simulink model "cont"  (R2017b)
settings: Solver=ode4  StartTime=0.0  StopTime=20  FixedStep=0.0001  RelTol=1e-3
settings Model: Creator=user  LastModifiedBy=user

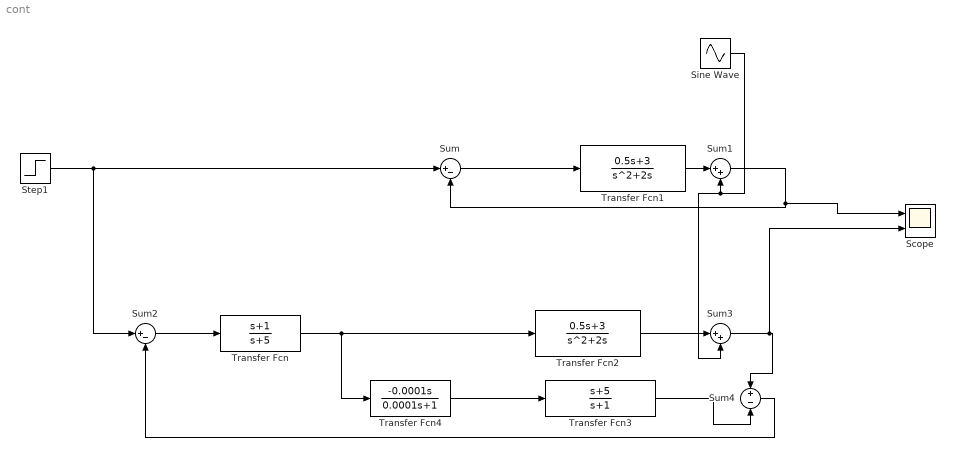
== system cont ==
  Scope : Scope  NumInputPorts=2
  Sine Wave : Sin  Amplitude=0.1  Frequency=10  Phase=2.7  SampleTime=0
  Step1 : Step  Time=0  SampleTime=0
  Sum : Sum  Inputs=|+-
  Sum1 : Sum  Inputs=|++
  Sum2 : Sum  Inputs=|+-
  Sum3 : Sum  Inputs=|++
  Sum4 : Sum  Inputs=+-
  Transfer Fcn : TransferFcn  Numerator=[1 1]  Denominator=[1 5]
  Transfer Fcn1 : TransferFcn  Numerator=[0.5 3]  Denominator=[1 2 0]
  Transfer Fcn2 : TransferFcn  Numerator=[0.5 3]  Denominator=[1 2 0]
  Transfer Fcn3 : TransferFcn  Numerator=[1 5]  Denominator=[1 1]
  Transfer Fcn4 : TransferFcn  Numerator=[-0.0001 0]  Denominator=[0.0001 1]
  wires:
  Sum/1 -> Transfer Fcn1/1
  Transfer Fcn1/1 -> Sum1/1
  Sine Wave/1 -> Sum3/2, Sum1/2
  Sum1/1 -> Scope/1, Sum/2
  Transfer Fcn2/1 -> Sum3/1
  Sum3/1 -> Scope/2, Sum4/1
  Step1/1 -> Sum/1, Sum2/1
  Sum4/1 -> Sum2/2
  Sum2/1 -> Transfer Fcn/1
  Transfer Fcn/1 -> Transfer Fcn4/1, Transfer Fcn2/1
  Transfer Fcn3/1 -> Sum4/2
  Transfer Fcn4/1 -> Transfer Fcn3/1
